simulink library "ddm"  (R2021b)
settings: Solver=VariableStepAuto  StartTime=0.0  StopTime=10.0  RelTol=1e-3
undefined symbols (not defined in the file or in its folder): ADDM_FrTMTqDev_X_Nm, ADDM_RrTMTqDev_X_Nm, ENUM_ADASACCSTA_ERROR, ENUM_ADASACCSTA_OFF, ENUM_ADASACCSTA_STANDBY, ENUM_ALLOWMOV_ALLOWREADY, ENUM_APS, ENUM_BRKSTA_ERROR, ENUM_BRKSTA_OFF, ENUM_BRKSTA_ON, ENUM_BRKSW_INVALID, ENUM_BRKSW_OFF, ENUM_BRKSW_ON, ENUM_CHGPREACTERRSTA_OBCPRE, ENUM_DCDCFAULTSTA_ANYFAULTLV1, ENUM_DCDCFAULTSTA_ANYFAULTLV2, ENUM_DRIVETRAIN_AWD, ENUM_DRIVETRAIN_FWD, ENUM_DRIVETRAIN_RWD, ENUM_EDUDRTSTA_NORMAL, ENUM_EPBSTA_APPLIED, ENUM_EPBSTA_RELEASED, ENUM_GEARACTUALPOSN_INVALID, ENUM_GEARACTUALPOSN_P, ENUM_HVBATTREADYPRE_READY, ENUM_MCUWARN_LV0, ENUM_MCUWARN_LV1, ENUM_MCUWARN_LV2, ENUM_MCUWARN_LV3, ENUM_MCUWARN_NOERROR, ENUM_OBCFAULTSTA_ANYFAULT, ENUM_PAS_R2F2, ENUM_PDFAULT_BATTPDFAIL, ENUM_PDFAULT_DCDCDISABLE, ENUM_PDFAULT_MCUDISABLE, ENUM_PDFAULT_MCUDISCHRG, ENUM_POWERSTA_OFF, ENUM_POWERSTA_ON, ENUM_POWERSTA_READY, ENUM_POWERSTA_STANDBY, ENUM_PRESSINDI_LOW, ENUM_PUFAULT_BATTUPFAIL, ENUM_PUFAULT_DCDCENABLEFAIL, ENUM_PUFAULT_PRECHRGCHKFAIL, ENUM_PUFAULT_SAFETYCHKFAIL, ENUM_PUSTATE_COMPLETED, ENUM_PWRSTASW_OFF, ENUM_PWRSTASW_OFFA, ENUM_PWRSTASW_OFFCHVCHRG, ENUM_PWRSTASW_OFFCLVCHRG, ENUM_PWRSTASW_ON, ENUM_PWRSTASW_ONHVCHRG, ENUM_PWRSTASW_READY, ENUM_PWRSTASW_STANDBY, ENUM_SHIFTCOMMAND_P, ENUM_SHIFTERERRSTA_PBUTTONFAILURE, ENUM_VEHMALFUNLV_2ND, ENUM_VEHMALFUNLV_3RD, ENUM_VEHMALFUNLV_4TH, ENUM_VEHMALFUNLV_NORMAL ... (+459)
libraries: hcu_lib x515, simulink x3
(part 4 of 25)

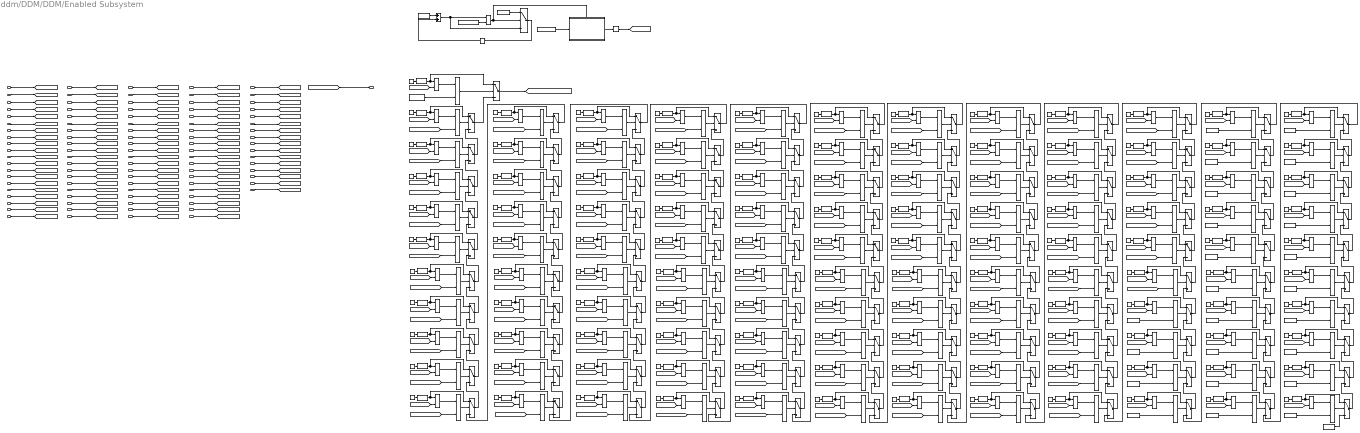
== system ddm/DDM/DDM/Enabled Subsystem ==
  VDDM_5vAPS1OoRCFS_flg : Inport
  VDDM_5vAPS2OoRCFS_flg : Inport  Port=2
  VDDM_BMSRdyCFS_flg : Inport  Port=3
  VDDM_BrkSWErrCFS_flg : Inport  Port=4
  VDDM_BrkSWNoBacCFS_flg : Inport  Port=5
  VDDM_C1ABM1CSCFS_flg : Inport  Port=6
  VDDM_C1ABM1LCCFS_flg : Inport  Port=7
  VDDM_C1ABM1RCCFS_flg : Inport  Port=8
  VDDM_C3BMS1CSCFS_flg : Inport  Port=9
  VDDM_C3BMS1LCCFS_flg : Inport  Port=10
  VDDM_C3BMS1RCCFS_flg : Inport  Port=11
  VDDM_C3BMS6CSCFS_flg : Inport  Port=12
  VDDM_C3BMS6LCCFS_flg : Inport  Port=13
  VDDM_C3BMS6RCCFS_flg : Inport  Port=14
  VDDM_C3CCU1CSCFS_flg : Inport  Port=15
  VDDM_C3CCU1LCCFS_flg : Inport  Port=16
  VDDM_C3CCU1RCCFS_flg : Inport  Port=17
  VDDM_C3CCU2CSCFS_flg : Inport  Port=18
  VDDM_C3CCU2LCCFS_flg : Inport  Port=19
  VDDM_C3CCU2RCCFS_flg : Inport  Port=20
  VDDM_DCDC4PreCFS_flg : Inport  Port=21
  VDDM_DCDCDisCFS_flg : Inport  Port=22
  VDDM_DCDCEnaCFS_flg : Inport  Port=23
  VDDM_DrStSWCFS_flg : Inport  Port=24
  VDDM_EPBLockTOCFS_flg : Inport  Port=25
  VDDM_EPBUnlockTOCFS_flg : Inport  Port=26
  VDDM_ESC1CSErrCFS_flg : Inport  Port=27
  VDDM_ESC1NoComCFS_flg : Inport  Port=28
  VDDM_ESC1RCErrCFS_flg : Inport  Port=29
  VDDM_ESC5CSErrCFS_flg : Inport  Port=30
  VDDM_ESC5NoComCFS_flg : Inport  Port=31
  VDDM_ESC5RCErrCFS_flg : Inport  Port=32
  VDDM_FLDoorSWCFS_flg : Inport  Port=33
  VDDM_FRDoorSWCFS_flg : Inport  Port=34
  VDDM_HVB4PreCFS_flg : Inport  Port=35
  VDDM_HVRlyCloCFS_flg : Inport  Port=36
  VDDM_HVRlyOpCFS_flg : Inport  Port=37
  VDDM_HiLvSaChkCFS_flg : Inport  Port=38
  VDDM_IniLVLoCFS_flg : Inport  Port=39
  VDDM_KeyAuthCFS_flg : Inport  Port=40
  VDDM_LVInErrCFS_flg : Inport  Port=41
  VDDM_LVSupHiCFS_flg : Inport  Port=42
  VDDM_LVSupLoCFS_flg : Inport  Port=43
  VDDM_Lv1ErrCFS_flg : Inport  Port=44
  VDDM_Lv2ErrCFS_flg : Inport  Port=45
  VDDM_Lv3ErrCFS_flg : Inport  Port=46
  VDDM_Lv4ErrCFS_flg : Inport  Port=47
  VDDM_MCU4PreCFS_flg : Inport  Port=48
  VDDM_MCUActCFS_flg : Inport  Port=49
  VDDM_MCUDisCFS_flg : Inport  Port=50
  VDDM_MCUNF1CSErrCFS_flg : Inport  Port=51
  VDDM_MCUNF1NoComCFS_flg : Inport  Port=52
  VDDM_MCUNF1RCErrCFS_flg : Inport  Port=53
  VDDM_MCUNR1CSErrCFS_flg : Inport  Port=54
  VDDM_MCUNR1NoComCFS_flg : Inport  Port=55
  VDDM_MCUNR1RCErrCFS_flg : Inport  Port=56
  VDDM_MidLvSaChkCFS_flg : Inport  Port=57
  VDDM_OBC4PreCFS_flg : Inport  Port=58
  VDDM_ONtoRdyCFS_flg : Inport  Port=59
  VDDM_RLDoorSWCFS_flg : Inport  Port=60
  VDDM_RRDoorSWCFS_flg : Inport  Port=61
  VDDM_Shifter1CSErrCFS_flg : Inport  Port=62
  VDDM_Shifter1NoComCFS_flg : Inport  Port=63
  VDDM_Shifter1RCErrCFS_flg : Inport  Port=64
  VDDM_HoodSWCFS_flg : Inport  Port=65
  VDDM_TailgaSWCFS_flg : Inport  Port=66
  VINP_ZoneDrMalfunLevel_enum : Inport  Port=67
  ZoneFrMalfunLevel_enum : Inport  Port=68
  VDDM_APS1SigOoRCFS_flg : Inport  Port=69
  VDDM_APS2SigOoRCFS_flg : Inport  Port=70
  VDDM_APSCorrErrCFS_flg : Inport  Port=71
  VDDM_FCM1NoComCFS_flg : Inport  Port=72
  VDDM_FCM1RCErrCFS_flg : Inport  Port=73
  VDDM_FCM1CSErrCFS_flg : Inport  Port=74
  VDDM_BMSSigErrCFS_flg : Inport  Port=75
  VDDM_FCMACCSigErrCFS_flg : Inport  Port=76
  VDDM_CCUSigErrCFS_flg : Inport  Port=77
  VDDM_ACCAccelCmdErrCFS_flg : Inport  Port=78
  VDDM_ESCSigErrCFS_flg : Inport  Port=79
  VDDM_ShifterSigErrCFS_flg : Inport  Port=80
  VDDM_DrVCUNoComCFS_flg : Inport  Port=81
  VDDM_FrVCUNoComCFS_flg : Inport  Port=82
  VDDM_ZoneDrSigErrCFS_flg : Inport  Port=83
  VDDM_ZoneFrSigErrCFS_flg : Inport  Port=84
  VDDM_EPS1NoComCFS_flg : Inport  Port=85
  VDDM_EPS1RCErrCFS_flg : Inport  Port=86
  VDDM_EPS1CSErrCFS_flg : Inport  Port=87
  VDDM_EPSSigErrCFS_flg : Inport  Port=88
  VDDM_FrMCUSigErrCFS_flg : Inport  Port=89
  VDDM_RrMCUSigErrCFS_flg : Inport  Port=90
  VDDM_EPB1NoComCFS_flg : Inport  Port=91
  VDDM_EPB1RCErrCFS_flg : Inport  Port=92
  VDDM_EPB1CSErrCFS_flg : Inport  Port=93
  VDDM_EPBSigErrCFS_flg : Inport  Port=94
  VDDM_FrMCUNTqErrCFS_flg : Inport  Port=95
  VDDM_RrMCUNTqErrCFS_flg : Inport  Port=96
  Add : Sum
  Constant : Constant  Value=ZERO_INT
  Constant1 : Constant  Value=ONE_INT
  Constant10 : Constant  Value=6  OutDataTypeStr=single
  Constant100 : Constant  Value=92  OutDataTypeStr=single
  Constant101 : Constant  Value=93  OutDataTypeStr=single
  Constant102 : Constant  Value=94  OutDataTypeStr=single
  Constant103 : Constant  Value=91  OutDataTypeStr=single
  Constant104 : Constant  Value=95  OutDataTypeStr=single
  Constant105 : Constant  Value=102  OutDataTypeStr=single
  Constant106 : Constant  Value=103  OutDataTypeStr=single
  Constant107 : Constant  Value=104  OutDataTypeStr=single
  Constant108 : Constant  Value=101  OutDataTypeStr=single
  Constant109 : Constant  Value=105  OutDataTypeStr=single
  Constant11 : Constant  Value=7  OutDataTypeStr=single
  Constant110 : Constant  Value=106  OutDataTypeStr=single
  Constant111 : Constant  Value=107  OutDataTypeStr=single
  Constant112 : Constant  Value=108  OutDataTypeStr=single
  Constant113 : Constant  Value=109  OutDataTypeStr=single
  Constant114 : Constant  Value=110  OutDataTypeStr=single
  Constant115 : Constant  Value=112  OutDataTypeStr=single
  Constant116 : Constant  Value=113  OutDataTypeStr=single
  Constant117 : Constant  Value=114  OutDataTypeStr=single
  Constant118 : Constant  Value=111  OutDataTypeStr=single
  Constant119 : Constant  Value=115  OutDataTypeStr=single
  Constant12 : Constant  Value=8  OutDataTypeStr=single
  Constant120 : Constant  Value=116  OutDataTypeStr=single
  Constant121 : Constant  Value=117  OutDataTypeStr=single
  Constant122 : Constant  Value=118  OutDataTypeStr=single
  Constant123 : Constant  Value=119  OutDataTypeStr=single
  Constant124 : Constant  Value=120  OutDataTypeStr=single
  Constant{125..132,135..150} (24 alike) : Constant  Value=FALSE
  Constant13 : Constant  Value=9  OutDataTypeStr=single
  Constant133 : Constant  Value=ZERO_INT
  Constant134 : Constant  Value=KDDM_DTCClockerMax_cnt
  Constant14 : Constant  Value=10  OutDataTypeStr=single
  Constant15 : Constant  Value=16  OutDataTypeStr=single
  Constant16 : Constant  Value=17  OutDataTypeStr=single
  Constant17 : Constant  Value=18  OutDataTypeStr=single
  Constant18 : Constant  Value=19  OutDataTypeStr=single
  Constant19 : Constant  Value=20  OutDataTypeStr=single
  Constant2 : Constant  Value=2  OutDataTypeStr=single
  Constant20 : Constant  Value=12  OutDataTypeStr=single
  Constant21 : Constant  Value=13  OutDataTypeStr=single
  Constant22 : Constant  Value=14  OutDataTypeStr=single
  Constant23 : Constant  Value=11  OutDataTypeStr=single
  Constant24 : Constant  Value=15  OutDataTypeStr=single
  Constant25 : Constant  Value=26  OutDataTypeStr=single
  Constant26 : Constant  Value=27  OutDataTypeStr=single
  Constant27 : Constant  Value=28  OutDataTypeStr=single
  Constant28 : Constant  Value=29  OutDataTypeStr=single
  Constant29 : Constant  Value=30  OutDataTypeStr=single
  Constant3 : Constant  Value=3  OutDataTypeStr=single
  Constant30 : Constant  Value=22  OutDataTypeStr=single
  Constant31 : Constant  Value=23  OutDataTypeStr=single
  Constant32 : Constant  Value=24  OutDataTypeStr=single
  Constant33 : Constant  Value=21  OutDataTypeStr=single
  Constant34 : Constant  Value=25  OutDataTypeStr=single
  Constant35 : Constant  Value=36  OutDataTypeStr=single
  Constant36 : Constant  Value=37  OutDataTypeStr=single
  Constant37 : Constant  Value=38  OutDataTypeStr=single
  Constant38 : Constant  Value=39  OutDataTypeStr=single
  Constant39 : Constant  Value=40  OutDataTypeStr=single
  Constant4 : Constant  Value=TRUE
  Constant40 : Constant  Value=32  OutDataTypeStr=single
  Constant41 : Constant  Value=33  OutDataTypeStr=single
  Constant42 : Constant  Value=34  OutDataTypeStr=single
  Constant43 : Constant  Value=31  OutDataTypeStr=single
  Constant44 : Constant  Value=35  OutDataTypeStr=single
  Constant45 : Constant  Value=46  OutDataTypeStr=single
  Constant46 : Constant  Value=47  OutDataTypeStr=single
  Constant47 : Constant  Value=48  OutDataTypeStr=single
  Constant48 : Constant  Value=49  OutDataTypeStr=single
  Constant49 : Constant  Value=50  OutDataTypeStr=single
  Constant5 : Constant  Value=KDDM_DTCDelay_cnt
  Constant50 : Constant  Value=42  OutDataTypeStr=single
  Constant51 : Constant  Value=43  OutDataTypeStr=single
  Constant52 : Constant  Value=44  OutDataTypeStr=single
  Constant53 : Constant  Value=41  OutDataTypeStr=single
  Constant54 : Constant  Value=45  OutDataTypeStr=single
  Constant55 : Constant  Value=56  OutDataTypeStr=single
  Constant56 : Constant  Value=57  OutDataTypeStr=single
  Constant57 : Constant  Value=58  OutDataTypeStr=single
  Constant58 : Constant  Value=59  OutDataTypeStr=single
  Constant59 : Constant  Value=60  OutDataTypeStr=single
  Constant6 : Constant  Value=4  OutDataTypeStr=single
  Constant60 : Constant  Value=52  OutDataTypeStr=single
  Constant61 : Constant  Value=53  OutDataTypeStr=single
  Constant62 : Constant  Value=54  OutDataTypeStr=single
  Constant63 : Constant  Value=51  OutDataTypeStr=single
  Constant64 : Constant  Value=55  OutDataTypeStr=single
  Constant65 : Constant  Value=66  OutDataTypeStr=single
  Constant66 : Constant  Value=67  OutDataTypeStr=single
  Constant67 : Constant  Value=68  OutDataTypeStr=single
  Constant68 : Constant  Value=69  OutDataTypeStr=single
  Constant69 : Constant  Value=70  OutDataTypeStr=single
  Constant7 : Constant  OutDataTypeStr=single
  Constant70 : Constant  Value=62  OutDataTypeStr=single
  Constant71 : Constant  Value=63  OutDataTypeStr=single
  Constant72 : Constant  Value=64  OutDataTypeStr=single
  Constant73 : Constant  Value=61  OutDataTypeStr=single
  Constant74 : Constant  Value=65  OutDataTypeStr=single
  Constant75 : Constant  Value=76  OutDataTypeStr=single
  Constant76 : Constant  Value=77  OutDataTypeStr=single
  Constant77 : Constant  Value=78  OutDataTypeStr=single
  Constant78 : Constant  Value=79  OutDataTypeStr=single
  Constant79 : Constant  Value=80  OutDataTypeStr=single
  Constant8 : Constant  Value=5  OutDataTypeStr=single
  Constant80 : Constant  Value=72  OutDataTypeStr=single
  Constant81 : Constant  Value=73  OutDataTypeStr=single
  Constant82 : Constant  Value=74  OutDataTypeStr=single
  Constant83 : Constant  Value=71  OutDataTypeStr=single
  Constant84 : Constant  Value=75  OutDataTypeStr=single
  Constant85 : Constant  Value=86  OutDataTypeStr=single
  Constant86 : Constant  Value=87  OutDataTypeStr=single
  Constant87 : Constant  Value=88  OutDataTypeStr=single
  Constant88 : Constant  Value=89  OutDataTypeStr=single
  Constant89 : Constant  Value=90  OutDataTypeStr=single
  Constant9 : Constant  Value=0  OutDataTypeStr=uint8
  Constant90 : Constant  Value=82  OutDataTypeStr=single
  Constant91 : Constant  Value=83  OutDataTypeStr=single
  Constant92 : Constant  Value=84  OutDataTypeStr=single
  Constant93 : Constant  Value=81  OutDataTypeStr=single
  Constant94 : Constant  Value=85  OutDataTypeStr=single
  Constant95 : Constant  Value=96  OutDataTypeStr=single
  Constant96 : Constant  Value=97  OutDataTypeStr=single
  Constant97 : Constant  Value=98  OutDataTypeStr=single
  Constant98 : Constant  Value=99  OutDataTypeStr=single
  Constant99 : Constant  Value=100  OutDataTypeStr=single
  Data Type Conversion{,1..120} (121 alike) : DataTypeConversion  OutDataTypeStr=uint8
  Delay : Delay  DelayLength=1
  IC : InitialCondition  Value=0
  Logical Operator{,1..120} (121 alike) : Logic  AllPortsSameDT=off  OutDataTypeStr=boolean
  Relational Operator : RelationalOperator  Operator=>  OutDataTypeStr=boolean  RndMeth=Simplest
  Relational Operator{1..121} (121 alike) : RelationalOperator  Operator===  OutDataTypeStr=boolean  RndMeth=Simplest
  Subsystem : Subsystem
  Switch{,1..121} (122 alike) : Switch  Criteria=u2 > Threshold
  VDDM_DTCDetect_enum : Outport
  wires:
  Constant1/1 -> Add/1
  IC/1 -> [DTC_clocker]
  Constant/1 -> Switch/1
  Subsystem/1(VDDM_DTCCounter_cnt) -> IC/1
  Add/1 -> Relational Operator/1, Switch/3
  Switch/1 -> Delay/1
  Delay/1 -> Add/2
  Constant134/1 -> Subsystem/1(KDDM_DTCClockerMax_cnt)
  Relational Operator/1 -> Switch/2, Subsystem/Trigger
  Constant5/1 -> Relational Operator/2
  Relational Operator13/1 -> Logical Operator20/1
  Constant16/1 -> Data Type Conversion18/1
  Switch1/1 -> [VDDM_DTCDetect_enum]  "VDDM_DTCDetect_enum"
  Relational Operator16/1 -> Logical Operator14/1
  [DTC_clocker] -> Relational Operator16/2
  Data Type Conversion16/1 -> Relational Operator18/1, Switch18/1
  Constant22/1 -> Data Type Conversion15/1
  Data Type Conversion18/1 -> Relational Operator20/1, Switch20/1
  Logical Operator16/1 -> Switch18/2
  Constant11/1 -> Data Type Conversion7/1
  Switch6/1 -> Switch5/3
  Switch16/1 -> Switch15/3
  [DTC_clocker] -> Relational Operator21/2
  Relational Operator14/1 -> Logical Operator12/1
  [VDDM_C3CCU2RCCFS_flg] -> Logical Operator12/2
  [DTC_clocker] -> Relational Operator19/2
  Relational Operator19/1 -> Logical Operator17/1
  Switch19/1 -> Switch18/3
  Constant20/1 -> Data Type Conversion13/1
  Constant15/1 -> Data Type Conversion17/1
  Logical Operator11/1 -> Switch14/2
  Switch15/1 -> Switch14/3
  Data Type Conversion6/1 -> Relational Operator7/1, Switch7/1
  [DTC_clocker] -> Relational Operator11/2
  [VDDM_C1ABM1LCCFS_flg] -> Logical Operator7/2
  Logical Operator10/1 -> Switch11/2
  [DTC_clocker] -> Relational Operator10/2
  Switch9/1 -> Switch8/3
  Switch10/1 -> Switch9/3
  Switch8/1 -> Switch7/3
  Logical Operator9/1 -> Switch10/2
  [DTC_clocker] -> Relational Operator7/2
  [DTC_clocker] -> Relational Operator5/2
  Switch3/1 -> Switch2/3
  [DTC_clocker] -> Relational Operator6/2
  Data Type Conversion4/1 -> Relational Operator5/1, Switch5/1
  Constant8/1 -> Data Type Conversion5/1
  Logical Operator/1 -> Switch2/2
  [DTC_clocker] -> Relational Operator1/2
  Relational Operator1/1 -> Logical Operator/1
  Data Type Conversion2/1 -> Relational Operator2/1, Switch3/1
  Constant4/1 -> Logical Operator1/2
  Logical Operator1/1 -> Switch1/2
  Data Type Conversion8/1 -> Relational Operator9/1, Switch9/1
  Relational Operator29/1 -> Logical Operator27/1
  Relational Operator27/1 -> Logical Operator25/1
  [VDDM_EPBUnlockTOCFS_flg] -> Logical Operator27/2
  Switch26/1 -> Switch25/3
  [DTC_clocker] -> Relational Operator29/2
  Switch7/1 -> Switch6/3
  Switch28/1 -> Switch27/3
  Data Type Conversion28/1 -> Relational Operator30/1, Switch30/1
  Switch22/1 -> Switch31/3
  Constant27/1 -> Data Type Conversion29/1
  Constant26/1 -> Data Type Conversion28/1
  Data Type Conversion15/1 -> Relational Operator17/1, Switch17/1
  Logical Operator26/1 -> Switch28/2
  [VDDM_C3BMS6LCCFS_flg] -> Logical Operator14/2
  Switch14/1 -> Switch11/3
  Relational Operator32/1 -> Logical Operator31/1
  Switch63/1 -> Switch62/3
  [VDDM_MCUNR1NoComCFS_flg] -> Logical Operator56/2
  Relational Operator59/1 -> Logical Operator57/1
  Data Type Conversion17/1 -> Relational Operator19/1, Switch19/1
  Relational Operator74/1 -> Logical Operator72/1
  Switch69/1 -> Switch68/3
  [DTC_clocker] -> Relational Operator47/2
  [DTC_clocker] -> Relational Operator76/2
  Relational Operator73/1 -> Logical Operator80/1
  Constant17/1 -> Data Type Conversion19/1
  Constant65/1 -> Data Type Conversion67/1
  [VDDM_FCM1NoComCFS_flg] -> Logical Operator73/2
  Switch74/1 -> Switch63/3
  [VDDM_C1ABM1RCCFS_flg] -> Logical Operator8/2
  [VDDM_ESC1RCErrCFS_flg] -> Logical Operator30/2
  Switch11/1 -> Switch10/3
  Data Type Conversion71/1 -> Relational Operator72/1, Switch74/1
  Relational Operator44/1 -> Logical Operator42/1
  Constant67/1 -> Data Type Conversion69/1
  Logical Operator3/1 -> Switch4/2
  [VDDM_MCUNF1CSErrCFS_flg] -> Logical Operator51/2
  Data Type Conversion58/1 -> Relational Operator60/1, Switch60/1
  Constant71/1 -> Data Type Conversion64/1
  Data Type Conversion66/1 -> Relational Operator68/1, Switch68/1
  Data Type Conversion23/1 -> Relational Operator25/1, Switch25/1
  Relational Operator24/1 -> Logical Operator22/1
  Relational Operator65/1 -> Logical Operator63/1
  Relational Operator71/1 -> Logical Operator69/1
  Logical Operator69/1 -> Switch71/2
  Switch62/1 -> Switch71/3
  Relational Operator70/1 -> Logical Operator68/1
  Switch65/1 -> Switch64/3
  Data Type Conversion53/1 -> Relational Operator55/1, Switch55/1
  [DTC_clocker] -> Relational Operator30/2
  Data Type Conversion12/1 -> Relational Operator14/1, Switch13/1
  [VINP_ZoneDrMalfunLevel_enum] -> Logical Operator68/2
  Constant73/1 -> Data Type Conversion61/1
  Relational Operator63/1 -> Logical Operator70/1
  Data Type Conversion51/1 -> Relational Operator52/1, Switch54/1
  Data Type Conversion61/1 -> Relational Operator62/1, Switch64/1
  Constant28/1 -> Data Type Conversion30/1
  Logical Operator68/1 -> Switch70/2
  Constant63/1 -> Data Type Conversion51/1
  Logical Operator58/1 -> Switch60/2
  Constant82/1 -> Data Type Conversion75/1
  [VDDM_MCUNF1RCErrCFS_flg] -> Logical Operator54/2
  Constant74/1 -> Data Type Conversion66/1
  Logical Operator27/1 -> Switch29/2
  [DTC_clocker] -> Relational Operator58/2
  Logical Operator52/1 -> Switch53/2
  Data Type Conversion54/1 -> Relational Operator56/1, Switch56/1
  Logical Operator54/1 -> Switch56/2
  Constant48/1 -> Data Type Conversion50/1
  Logical Operator60/1 -> Switch52/2
  Constant19/1 -> Data Type Conversion12/1
  Data Type Conversion26/1 -> Relational Operator28/1, Switch28/1
  [VDDM_HiLvSaChkCFS_flg] -> Logical Operator39/2
  [DTC_clocker] -> Relational Operator8/2
  Relational Operator57/1 -> Logical Operator55/1
  Switch31/1 -> Switch30/3
  [DTC_clocker] -> Relational Operator54/2
  [DTC_clocker] -> Relational Operator49/2
  [DTC_clocker] -> Relational Operator17/2
  Logical Operator47/1 -> Switch49/2
  Data Type Conversion41/1 -> Relational Operator42/1, Switch44/1
  [DTC_clocker] -> Relational Operator51/2
  [VDDM_LVInErrCFS_flg] -> Logical Operator41/2
  Relational Operator50/1 -> Logical Operator48/1
  Constant45/1 -> Data Type Conversion47/1
  Relational Operator6/1 -> Logical Operator5/1
  Switch80/1 -> Switch79/3
  [DTC_clocker] -> Relational Operator50/2
  Logical Operator2/1 -> Switch3/2
  Data Type Conversion43/1 -> Relational Operator45/1, Switch45/1
  Constant51/1 -> Data Type Conversion44/1
  Logical Operator17/1 -> Switch19/2
  Logical Operator64/1 -> Switch66/2
  Switch44/1 -> Switch33/3
  Switch42/1 -> Switch51/3
  Constant52/1 -> Data Type Conversion45/1
  Constant3/1 -> Data Type Conversion3/1
  Data Type Conversion44/1 -> Relational Operator46/1, Switch46/1
  Switch46/1 -> Switch45/3
  Constant49/1 -> Data Type Conversion42/1
  [VDDM_APS2SigOoRCFS_flg] -> Logical Operator62/2
  [VDDM_MCUActCFS_flg] -> Logical Operator50/2
  Logical Operator44/1 -> Switch46/2
  [VDDM_LVSupLoCFS_flg] -> Logical Operator44/2
  [DTC_clocker] -> Relational Operator66/2
  Relational Operator48/1 -> Logical Operator46/1
  Data Type Conversion7/1 -> Relational Operator8/1, Switch8/1
  [DTC_clocker] -> Relational Operator45/2
  [VDDM_C3CCU1CSCFS_flg] -> Logical Operator16/2
  [VDDM_MCUDisCFS_flg] -> Logical Operator42/2
  Constant18/1 -> Data Type Conversion20/1
  Data Type Conversion32/1 -> Relational Operator34/1, Switch33/1
  Data Type Conversion19/1 -> Relational Operator21/1, Switch21/1
  Constant2/1 -> Data Type Conversion2/1
  Switch50/1 -> Switch49/3
  [VDDM_OBC4PreCFS_flg] -> Logical Operator59/2
  [DTC_clocker] -> Relational Operator32/2
  Logical Operator46/1 -> Switch48/2
  [VDDM_ESC1CSErrCFS_flg] -> Logical Operator28/2
  Constant78/1 -> Data Type Conversion80/1
  [DTC_clocker] -> Relational Operator36/2
  [VDDM_HVRlyOpCFS_flg] -> Logical Operator38/2
  Data Type Conversion39/1 -> Relational Operator41/1, Switch41/1
  Logical Operator32/1 -> Switch33/2
  Constant41/1 -> Data Type Conversion34/1
  Constant47/1 -> Data Type Conversion49/1
  Logical Operator22/1 -> Switch23/2
  Logical Operator40/1 -> Switch32/2
  Relational Operator34/1 -> Logical Operator32/1
  Logical Operator45/1 -> Switch47/2
  Constant36/1 -> Data Type Conversion38/1
  Data Type Conversion50/1 -> Relational Operator43/1, Switch42/1
  Relational Operator38/1 -> Logical Operator36/1
  Constant44/1 -> Data Type Conversion36/1
  Data Type Conversion42/1 -> Relational Operator44/1, Switch43/1
  Constant37/1 -> Data Type Conversion39/1
  [DTC_clocker] -> Relational Operator43/2
  Constant38/1 -> Data Type Conversion40/1
  Switch39/1 -> Switch38/3
  Constant6/1 -> Data Type Conversion4/1
  Logical Operator35/1 -> Switch37/2
  Logical Operator39/1 -> Switch41/2
  [DTC_clocker] -> Relational Operator72/2
  [DTC_clocker] -> Relational Operator40/2
  Switch32/1 -> Switch41/3
  [VDDM_MCU4PreCFS_flg] -> Logical Operator49/2
  Data Type Conversion3/1 -> Relational Operator4/1, Switch4/1
  Constant25/1 -> Data Type Conversion27/1
  Data Type Conversion33/1 -> Relational Operator35/1, Switch35/1
  Logical Operator31/1 -> Switch34/2
  Switch45/1 -> Switch44/3
  Switch5/1 -> Switch4/3
  Logical Operator20/1 -> Switch12/2
  [DTC_clocker] -> Relational Operator27/2
  Switch27/1 -> Switch26/3
  [DTC_clocker] -> Relational Operator37/2
  [DTC_clocker] -> Relational Operator41/2
  Relational Operator36/1 -> Logical Operator34/1
  [VDDM_ESC5RCErrCFS_flg] -> Logical Operator33/2
  Switch101/1 -> Switch100/3
  [DTC_clocker] -> Relational Operator92/2
  [VDDM_Shifter1CSErrCFS_flg] -> Logical Operator63/2
  Relational Operator52/1 -> Logical Operator51/1
  Logical Operator94/1 -> Switch96/2
  [DTC_clocker] -> Relational Operator101/2
  [VDDM_EPBSigErrCFS_flg] -> Logical Operator95/2
  Constant69/1 -> Data Type Conversion62/1
  Relational Operator83/1 -> Logical Operator90/1
  [DTC_clocker] -> Relational Operator70/2
  Data Type Conversion100/1 -> Relational Operator93/1, Switch92/1
  [DTC_clocker] -> Relational Operator94/2
  Data Type Conversion57/1 -> Relational Operator59/1, Switch59/1
  Data Type Conversion20/1 -> Relational Operator13/1, Switch12/1
  Relational Operator49/1 -> Logical Operator47/1
  Switch53/1 -> Switch52/3
  [VDDM_RrMCUNTqErrCFS_flg] -> Logical Operator97/2
  Relational Operator95/1 -> Logical Operator93/1
  Constant88/1 -> Data Type Conversion90/1
  Relational Operator101/1 -> Logical Operator99/1
  [VDDM_RRDoorSWCFS_flg] -> Logical Operator61/2
  Constant23/1 -> Data Type Conversion11/1
  Relational Operator94/1 -> Logical Operator92/1
  Switch54/1 -> Switch43/3
  [DTC_clocker] -> Relational Operator63/2
  [DTC_clocker] -> Relational Operator42/2
  [DTC_clocker] -> Relational Operator98/2
  Logical Operator4/1 -> Switch5/2
  Logical Operator92/1 -> Switch93/2
  Data Type Conversion/1 -> Relational Operator3/1, Switch1/1
  Relational Operator92/1 -> Logical Operator91/1
  Constant98/1 -> Data Type Conversion100/1
  Logical Operator33/1 -> Switch35/2
  Switch48/1 -> Switch47/3
  Data Type Conversion81/1 -> Relational Operator82/1, Switch84/1
  Constant101/1 -> Data Type Conversion94/1
  Constant54/1 -> Data Type Conversion46/1
  Data Type Conversion84/1 -> Relational Operator86/1, Switch86/1
  Switch94/1 -> Switch83/3
  [DTC_clocker] -> Relational Operator56/2
  Constant13/1 -> Data Type Conversion9/1
  Constant85/1 -> Data Type Conversion87/1
  Switch23/1 -> Switch22/3
  [DTC_clocker] -> Relational Operator26/2
  Switch92/1 -> Switch101/3
  Switch89/1 -> Switch88/3
  Data Type Conversion73/1 -> Relational Operator75/1, Switch75/1
  [VDDM_HVRlyCloCFS_flg] -> Logical Operator37/2
  Data Type Conversion27/1 -> Relational Operator29/1, Switch29/1
  Logical Operator86/1 -> Switch88/2
  Constant81/1 -> Data Type Conversion74/1
  Data Type Conversion14/1 -> Relational Operator16/1, Switch16/1
  [VDDM_ONtoRdyCFS_flg] -> Logical Operator60/2
  Switch71/1 -> Switch70/3
  Switch87/1 -> Switch86/3
  [DTC_clocker] -> Relational Operator85/2
  Data Type Conversion70/1 -> Relational Operator63/1, Switch62/1
  Relational Operator82/1 -> Logical Operator81/1
  Logical Operator83/1 -> Switch85/2
  Relational Operator78/1 -> Logical Operator76/1
  [DTC_clocker] -> Relational Operator86/2
  Data Type Conversion35/1 -> Relational Operator37/1, Switch37/1
  Relational Operator12/1 -> Logical Operator11/1
  Constant56/1 -> Data Type Conversion58/1
  Constant90/1 -> Data Type Conversion83/1
  Relational Operator15/1 -> Logical Operator13/1
  Data Type Conversion82/1 -> Relational Operator84/1, Switch83/1
  [VDDM_MCUNF1NoComCFS_flg] -> Logical Operator53/2
  [VDDM_DCDC4PreCFS_flg] -> Logical Operator21/2
  Constant93/1 -> Data Type Conversion81/1
  Logical Operator55/1 -> Switch57/2
  Data Type Conversion93/1 -> Relational Operator95/1, Switch95/1
  Switch83/1 -> Switch82/3
  Logical Operator85/1 -> Switch87/2
  [DTC_clocker] -> Relational Operator69/2
  Switch29/1 -> Switch28/3
  Switch70/1 -> Switch69/3
  Constant87/1 -> Data Type Conversion89/1
  [DTC_clocker] -> Relational Operator84/2
  [DTC_clocker] -> Relational Operator87/2
  Switch38/1 -> Switch37/3
  Relational Operator11/1 -> Logical Operator10/1
  Relational Operator4/1 -> Logical Operator3/1
  Logical Operator88/1 -> Switch90/2
  Logical Operator76/1 -> Switch78/2
  Switch78/1 -> Switch77/3
  Relational Operator88/1 -> Logical Operator86/1
  Relational Operator89/1 -> Logical Operator87/1
  Switch43/1 -> Switch42/3
  Data Type Conversion34/1 -> Relational Operator36/1, Switch36/1
  [DTC_clocker] -> Relational Operator81/2
  [VDDM_EPS1NoComCFS_flg] -> Logical Operator86/2
  Relational Operator10/1 -> Logical Operator9/1
  Relational Operator72/1 -> Logical Operator71/1
  Relational Operator55/1 -> Logical Operator53/1
  Switch52/1 -> Switch61/3
  Constant39/1 -> Data Type Conversion32/1
  [VDDM_FrMCUNTqErrCFS_flg] -> Logical Operator96/2
  Constant89/1 -> Data Type Conversion82/1
  Logical Operator49/1 -> Switch51/2
  [VDDM_EPS1RCErrCFS_flg] -> Logical Operator87/2
  Relational Operator17/1 -> Logical Operator15/1
  Logical Operator6/1 -> Switch7/2
  [VDDM_FLDoorSWCFS_flg] -> Logical Operator34/2
  Relational Operator18/1 -> Logical Operator16/1
  [DTC_clocker] -> Relational Operator75/2
  Constant40/1 -> Data Type Conversion33/1
  Data Type Conversion68/1 -> Relational Operator70/1, Switch70/1
  [VDDM_ESCSigErrCFS_flg] -> Logical Operator80/2
  [DTC_clocker] -> Relational Operator59/2
  Constant75/1 -> Data Type Conversion77/1
  Data Type Conversion72/1 -> Relational Operator74/1, Switch73/1
  [VDDM_MCUNR1RCErrCFS_flg] -> Logical Operator57/2
  Data Type Conversion74/1 -> Relational Operator76/1, Switch76/1
  Switch88/1 -> Switch87/3
  [DTC_clocker] -> Relational Operator12/2
  [DTC_clocker] -> Relational Operator77/2
  [DTC_clocker] -> Relational Operator74/2
  Relational Operator111/1 -> Logical Operator108/1
  Switch68/1 -> Switch67/3
  Switch49/1 -> Switch48/3
  Constant147/1 -> Logical Operator109/2
  Relational Operator9/1 -> Logical Operator8/1
  [DTC_clocker] -> Relational Operator95/2
  Logical Operator105/1 -> Switch108/2
  Logical Operator77/1 -> Switch79/2
  [DTC_clocker] -> Relational Operator52/2
  Relational Operator102/1 -> Logical Operator109/1
  Relational Operator53/1 -> Logical Operator60/1
  [DTC_clocker] -> Relational Operator4/2
  Logical Operator62/1 -> Switch63/2
  Switch13/1 -> Switch12/3
  [VDDM_FrMCUSigErrCFS_flg] -> Logical Operator90/2
  Constant140/1 -> Logical Operator104/2
  Logical Operator75/1 -> Switch77/2
  Constant76/1 -> Data Type Conversion78/1
  Data Type Conversion65/1 -> Relational Operator67/1, Switch67/1
  [VDDM_C3CCU2LCCFS_flg] -> Logical Operator20/2
  [VDDM_DCDCDisCFS_flg] -> Logical Operator23/2
  Switch73/1 -> Switch72/3
  Switch90/1 -> Switch89/3
  Relational Operator105/1 -> Logical Operator101/1
  Relational Operator69/1 -> Logical Operator67/1
  Switch56/1 -> Switch55/3
  Data Type Conversion21/1 -> Relational Operator22/1, Switch24/1
  [DTC_clocker] -> Relational Operator28/2
  [VDDM_RrMCUSigErrCFS_flg] -> Logical Operator82/2
  Relational Operator93/1 -> Logical Operator100/1
  [VDDM_RLDoorSWCFS_flg] -> Logical Operator52/2
  Switch34/1 -> Switch23/3
  Switch106/1 -> Switch93/3
  Constant60/1 -> Data Type Conversion53/1
  Relational Operator28/1 -> Logical Operator26/1
  [DTC_clocker] -> Relational Operator62/2
  Logical Operator19/1 -> Switch21/2
  Relational Operator77/1 -> Logical Operator75/1
  Constant7/1 -> Data Type Conversion1/1
  Logical Operator70/1 -> Switch62/2
  Data Type Conversion91/1 -> Relational Operator92/1, Switch94/1
  [VDDM_HoodSWCFS_flg] -> Logical Operator66/2
  Data Type Conversion52/1 -> Relational Operator54/1, Switch53/1
  Switch100/1 -> Switch99/3
  [DTC_clocker] -> Relational Operator13/2
  Logical Operator53/1 -> Switch55/2
  Constant100/1 -> Data Type Conversion93/1
  Data Type Conversion76/1 -> Relational Operator78/1, Switch78/1
  Logical Operator59/1 -> Switch61/2
  Constant14/1 -> Data Type Conversion10/1
  Logical Operator30/1 -> Switch22/2
  Constant94/1 -> Data Type Conversion86/1
  Logical Operator97/1 -> Switch99/2
  [DTC_clocker] -> Relational Operator88/2
  [VDDM_HVB4PreCFS_flg] -> Logical Operator36/2
  Relational Operator99/1 -> Logical Operator97/1
  Relational Operator100/1 -> Logical Operator98/1
  [DTC_clocker] -> Relational Operator68/2
  Constant68/1 -> Data Type Conversion70/1
  [VDDM_MCUNR1CSErrCFS_flg] -> Logical Operator55/2
  Logical Operator111/1 -> Switch114/2
  Relational Operator25/1 -> Logical Operator23/1
  Constant110/1 -> Data Type Conversion108/1
  [VDDM_EPBLockTOCFS_flg] -> Logical Operator26/2
  Switch79/1 -> Switch78/3
  Logical Operator109/1 -> Switch102/2
  Switch81/1 -> Switch80/3
  Relational Operator113/1 -> Logical Operator120/1
  [DTC_clocker] -> Relational Operator61/2
  [DTC_clocker] -> Relational Operator33/2
  Relational Operator90/1 -> Logical Operator88/1
  Relational Operator2/1 -> Logical Operator2/1
  Relational Operator120/1 -> Logical Operator117/1
  Constant123/1 -> Data Type Conversion111/1
  Data Type Conversion29/1 -> Relational Operator31/1, Switch31/1
  Logical Operator74/1 -> Switch76/2
  Data Type Conversion11/1 -> Relational Operator12/1, Switch14/1
  Logical Operator21/1 -> Switch24/2
  Relational Operator114/1 -> Logical Operator112/1
  Relational Operator41/1 -> Logical Operator39/1
  Relational Operator85/1 -> Logical Operator83/1
  Relational Operator35/1 -> Logical Operator33/1
  Constant122/1 -> Data Type Conversion120/1
  [DTC_clocker] -> Relational Operator46/2
  Relational Operator5/1 -> Logical Operator4/1
  Data Type Conversion49/1 -> Relational Operator51/1, Switch51/1
  Relational Operator119/1 -> Logical Operator116/1
  Data Type Conversion106/1 -> Relational Operator109/1, Switch109/1
  Constant33/1 -> Data Type Conversion21/1
  Logical Operator23/1 -> Switch25/2
  [VDDM_ESC5NoComCFS_flg] -> Logical Operator31/2
  [VDDM_ESC5CSErrCFS_flg] -> Logical Operator22/2
  Data Type Conversion80/1 -> Relational Operator73/1, Switch72/1
  Switch57/1 -> Switch56/3
  [DTC_clocker] -> Relational Operator99/2
  [VDDM_EPS1CSErrCFS_flg] -> Logical Operator88/2
  [VDDM_C3BMS1LCCFS_flg] -> Logical Operator10/2
  Constant43/1 -> Data Type Conversion31/1
  Switch82/1 -> Switch91/3
  Switch114/1 -> Switch113/3
  Logical Operator78/1 -> Switch80/2
  Logical Operator119/1 -> Switch112/2
  [VDDM_ShifterSigErrCFS_flg] -> Logical Operator72/2
  Relational Operator37/1 -> Logical Operator35/1
  Relational Operator98/1 -> Logical Operator96/1
  [DTC_clocker] -> Relational Operator113/2
  Constant117/1 -> Data Type Conversion116/1
  [VDDM_C1ABM1CSCFS_flg] -> Logical Operator6/2
  [VDDM_FCM1RCErrCFS_flg] -> Logical Operator74/2
  Constant128/1 -> Logical Operator118/2
  Relational Operator76/1 -> Logical Operator74/1
  Logical Operator120/1 -> Switch113/2
  Switch112/1 -> Switch121/3
  Data Type Conversion87/1 -> Relational Operator89/1, Switch89/1
  [VDDM_BrkSWErrCFS_flg] -> Logical Operator4/2
  Logical Operator93/1 -> Switch95/2
  [VDDM_C3BMS1CSCFS_flg] -> Logical Operator9/2
  Logical Operator90/1 -> Switch82/2
  Relational Operator103/1 -> Logical Operator110/1
  Switch33/1 -> Switch32/3
  Constant53/1 -> Data Type Conversion41/1
  Switch105/1 -> Switch104/3
  Relational Operator20/1 -> Logical Operator18/1
  Logical Operator37/1 -> Switch39/2
  Data Type Conversion55/1 -> Relational Operator57/1, Switch57/1
  Constant115/1 -> Data Type Conversion114/1
  Constant62/1 -> Data Type Conversion55/1
  Constant92/1 -> Data Type Conversion85/1
  Constant64/1 -> Data Type Conversion56/1
  Data Type Conversion98/1 -> Relational Operator100/1, Switch100/1
  Switch108/1 -> Switch107/3
  Constant126/1 -> Logical Operator116/2
  Switch107/1 -> Switch106/3
  [DTC_clocker] -> Relational Operator14/2
  Data Type Conversion109/1 -> Relational Operator102/1, Switch102/1
  Switch59/1 -> Switch58/3
  Switch18/1 -> Switch17/3
  Data Type Conversion38/1 -> Relational Operator40/1, Switch40/1
  Relational Operator30/1 -> Logical Operator28/1
  Relational Operator112/1 -> Logical Operator119/1
  [VDDM_BMSRdyCFS_flg] -> Logical Operator3/2
  [DTC_clocker] -> Relational Operator93/2
  Switch35/1 -> Switch34/3
  Logical Operator114/1 -> Switch117/2
  [DTC_clocker] -> Relational Operator97/2
  Data Type Conversion69/1 -> Relational Operator71/1, Switch71/1
  Logical Operator82/1 -> Switch83/2
  Logical Operator98/1 -> Switch100/2
  Data Type Conversion86/1 -> Relational Operator88/1, Switch88/1
  Constant141/1 -> Logical Operator114/2
  Constant137/1 -> Logical Operator100/2
  Switch60/1 -> Switch59/3
  Relational Operator45/1 -> Logical Operator43/1
  Data Type Conversion111/1 -> Relational Operator115/1, Switch114/1
  Switch41/1 -> Switch40/3
  Switch2/1 -> Switch1/3
  Constant12/1 -> Data Type Conversion8/1
  [VDDM_EPB1CSErrCFS_flg] -> Logical Operator94/2
  Data Type Conversion113/1 -> Relational Operator116/1, Switch115/1
  Data Type Conversion46/1 -> Relational Operator48/1, Switch48/1
  Data Type Conversion63/1 -> Relational Operator65/1, Switch65/1
  Data Type Conversion107/1 -> Relational Operator110/1, Switch110/1
  Constant119/1 -> Data Type Conversion117/1
  Logical Operator43/1 -> Switch45/2
  Logical Operator87/1 -> Switch89/2
  Data Type Conversion97/1 -> Relational Operator99/1, Switch99/1
  [VDDM_5vAPS1OoRCFS_flg] -> Logical Operator/2
  Constant58/1 -> Data Type Conversion60/1
  [DTC_clocker] -> Relational Operator31/2
  Data Type Conversion95/1 -> Relational Operator97/1, Switch97/1
  Switch67/1 -> Switch66/3
  Switch84/1 -> Switch73/3
  Relational Operator87/1 -> Logical Operator85/1
  Constant136/1 -> Logical Operator99/2
  [DTC_clocker] -> Relational Operator118/2
  Switch119/1 -> Switch118/3
  [DTC_clocker] -> Relational Operator83/2
  Relational Operator121/1 -> Logical Operator118/1
  Logical Operator24/1 -> Switch26/2
  Constant70/1 -> Data Type Conversion63/1
  Constant129/1 -> Logical Operator119/2
  Data Type Conversion102/1 -> Relational Operator104/1, Switch106/1
  Relational Operator62/1 -> Logical Operator61/1
  Relational Operator118/1 -> Logical Operator115/1
  Switch91/1 -> Switch90/3
  [VDDM_FrVCUNoComCFS_flg] -> Logical Operator83/2
  Switch113/1 -> Switch112/3
  Logical Operator28/1 -> Switch30/2
  Relational Operator46/1 -> Logical Operator44/1
  Data Type Conversion96/1 -> Relational Operator98/1, Switch98/1
  [DTC_clocker] -> Relational Operator79/2
  Constant42/1 -> Data Type Conversion35/1
  Data Type Conversion118/1 -> Relational Operator121/1, Switch121/1
  Data Type Conversion108/1 -> Relational Operator111/1, Switch111/1
  Constant10/1 -> Data Type Conversion6/1
  Logical Operator80/1 -> Switch72/2
  Relational Operator58/1 -> Logical Operator56/1
  Logical Operator117/1 -> Switch120/2
  Data Type Conversion25/1 -> Relational Operator27/1, Switch27/1
  [VDDM_Lv2ErrCFS_flg] -> Logical Operator46/2
  Relational Operator91/1 -> Logical Operator89/1
  Logical Operator104/1 -> Switch107/2
  Relational Operator21/1 -> Logical Operator19/1
  Switch20/1 -> Switch19/3
  [DTC_clocker] -> Relational Operator44/2
  Logical Operator66/1 -> Switch68/2
  Relational Operator117/1 -> Logical Operator114/1
  [DTC_clocker] -> Relational Operator82/2
  Data Type Conversion77/1 -> Relational Operator79/1, Switch79/1
  Data Type Conversion1/1 -> Relational Operator1/1, Switch2/1
  [VDDM_C3CCU2CSCFS_flg] -> Logical Operator19/2
  Switch61/1 -> Switch60/3
  Switch99/1 -> Switch98/3
  Data Type Conversion37/1 -> Relational Operator39/1, Switch39/1
  Logical Operator89/1 -> Switch91/2
  Constant131/1 -> Logical Operator111/2
  [VDDM_IniLVLoCFS_flg] -> Logical Operator40/2
  Relational Operator61/1 -> Logical Operator59/1
  Logical Operator61/1 -> Switch64/2
  Data Type Conversion110/1 -> Relational Operator103/1, Switch103/1
  Logical Operator79/1 -> Switch81/2
  [VDDM_ZoneDrSigErrCFS_flg] -> Logical Operator84/2
  [DTC_clocker] -> Relational Operator108/2
  Switch111/1 -> Switch110/3
  [DTC_clocker] -> Relational Operator23/2
  Logical Operator91/1 -> Switch94/2
  Logical Operator48/1 -> Switch50/2
  Switch75/1 -> Switch74/3
  Logical Operator25/1 -> Switch27/2
  [VDDM_DCDCEnaCFS_flg] -> Logical Operator24/2
  [DTC_clocker] -> Relational Operator116/2
  [ZoneFrMalfunLevel_enum] -> Logical Operator69/2
  Logical Operator101/1 -> Switch104/2
  [VDDM_APSCorrErrCFS_flg] -> Logical Operator71/2
  Logical Operator96/1 -> Switch98/2
  Switch58/1 -> Switch57/3
  [DTC_clocker] -> Relational Operator24/2
  Data Type Conversion30/1 -> Relational Operator23/1, Switch22/1
  Relational Operator109/1 -> Logical Operator106/1
  [DTC_clocker] -> Relational Operator65/2
  Data Type Conversion59/1 -> Relational Operator61/1, Switch61/1
  Relational Operator47/1 -> Logical Operator45/1
  [VDDM_Lv3ErrCFS_flg] -> Logical Operator47/2
  Logical Operator5/1 -> Switch6/2
  [VDDM_KeyAuthCFS_flg] -> Logical Operator32/2
  [DTC_clocker] -> Relational Operator104/2
  Constant29/1 -> Data Type Conversion22/1
  Constant99/1 -> Data Type Conversion92/1
  Constant121/1 -> Data Type Conversion119/1
  [DTC_clocker] -> Relational Operator120/2
  Constant66/1 -> Data Type Conversion68/1
  Logical Operator115/1 -> Switch118/2
  Relational Operator66/1 -> Logical Operator64/1
  Constant83/1 -> Data Type Conversion71/1
  Data Type Conversion13/1 -> Relational Operator15/1, Switch15/1
  Logical Operator71/1 -> Switch74/2
  [DTC_clocker] -> Relational Operator71/2
  [DTC_clocker] -> Relational Operator96/2
  Constant106/1 -> Data Type Conversion105/1
  [DTC_clocker] -> Relational Operator73/2
  [VDDM_C3CCU1LCCFS_flg] -> Logical Operator17/2
  Data Type Conversion117/1 -> Relational Operator120/1, Switch120/1
  [DTC_clocker] -> Relational Operator57/2
  [DTC_clocker] -> Relational Operator80/2
  Data Type Conversion45/1 -> Relational Operator47/1, Switch47/1
  [VDDM_C3BMS6RCCFS_flg] -> Logical Operator15/2
  Logical Operator118/1 -> Switch121/2
  Relational Operator22/1 -> Logical Operator21/1
  [DTC_clocker] -> Relational Operator105/2
  Logical Operator57/1 -> Switch59/2
  Relational Operator60/1 -> Logical Operator58/1
  Constant97/1 -> Data Type Conversion99/1
  Relational Operator26/1 -> Logical Operator24/1
  Data Type Conversion31/1 -> Relational Operator32/1, Switch34/1
  Switch21/1 -> Switch20/3
  [DTC_clocker] -> Relational Operator2/2
  Constant112/1 -> Data Type Conversion110/1
  Constant113/1 -> Data Type Conversion101/1
  [DTC_clocker] -> Relational Operator109/2
  Data Type Conversion75/1 -> Relational Operator77/1, Switch77/1
  Logical Operator12/1 -> Switch13/2
  [DTC_clocker] -> Relational Operator20/2
  Data Type Conversion67/1 -> Relational Operator69/1, Switch69/1
  Constant103/1 -> Data Type Conversion91/1
  Logical Operator29/1 -> Switch31/2
  Data Type Conversion88/1 -> Relational Operator90/1, Switch90/1
  [DTC_clocker] -> Relational Operator78/2
  [DTC_clocker] -> Relational Operator91/2
  [DTC_clocker] -> Relational Operator35/2
  Relational Operator7/1 -> Logical Operator6/1
  [VDDM_Shifter1RCErrCFS_flg] -> Logical Operator65/2
  Constant142/1 -> Logical Operator112/2
  Constant116/1 -> Data Type Conversion115/1
  Logical Operator51/1 -> Switch54/2
  Relational Operator40/1 -> Logical Operator38/1
  [VDDM_EPB1RCErrCFS_flg] -> Logical Operator93/2
  [VDDM_EPSSigErrCFS_flg] -> Logical Operator89/2
  Relational Operator54/1 -> Logical Operator52/1
  Relational Operator39/1 -> Logical Operator37/1
  Logical Operator42/1 -> Switch43/2
  [DTC_clocker] -> Relational Operator111/2
  Data Type Conversion104/1 -> Relational Operator107/1, Switch107/1
  [VDDM_EPB1NoComCFS_flg] -> Logical Operator91/2
  [VDDM_5vAPS2OoRCFS_flg] -> Logical Operator2/2
  Switch40/1 -> Switch39/3
  Constant111/1 -> Data Type Conversion109/1
  Constant50/1 -> Data Type Conversion43/1
  Logical Operator95/1 -> Switch97/2
  [DTC_clocker] -> Relational Operator102/2
  Logical Operator102/1 -> Switch106/2
  [DTC_clocker] -> Relational Operator90/2
  [DTC_clocker] -> Relational Operator67/2
  Data Type Conversion62/1 -> Relational Operator64/1, Switch63/1
  Data Type Conversion101/1 -> Relational Operator105/1, Switch104/1
  Constant91/1 -> Data Type Conversion84/1
  Logical Operator81/1 -> Switch84/2
  Constant143/1 -> Logical Operator105/2
  Logical Operator108/1 -> Switch111/2
  Constant107/1 -> Data Type Conversion106/1
  Constant104/1 -> Data Type Conversion96/1
  Constant96/1 -> Data Type Conversion98/1
  Switch12/1 -> Switch21/3
  [DTC_clocker] -> Relational Operator115/2
  [DTC_clocker] -> Relational Operator121/2
  Data Type Conversion48/1 -> Relational Operator50/1, Switch50/1
  [VDDM_CCUSigErrCFS_flg] -> Logical Operator78/2
  [VDDM_C3CCU1RCCFS_flg] -> Logical Operator18/2
  Constant150/1 -> Logical Operator103/2
  Logical Operator72/1 -> Switch73/2
  Constant84/1 -> Data Type Conversion76/1
  [DTC_clocker] -> Relational Operator39/2
  Constant109/1 -> Data Type Conversion107/1
  [VDDM_ZoneFrSigErrCFS_flg] -> Logical Operator85/2
  Logical Operator36/1 -> Switch38/2
  Logical Operator106/1 -> Switch109/2
  Constant46/1 -> Data Type Conversion48/1
  Logical Operator99/1 -> Switch101/2
  [VDDM_FRDoorSWCFS_flg] -> Logical Operator35/2
  Relational Operator116/1 -> Logical Operator113/1
  Constant77/1 -> Data Type Conversion79/1
  Logical Operator7/1 -> Switch8/2
  [DTC_clocker] -> Relational Operator22/2
  Constant24/1 -> Data Type Conversion16/1
  Constant86/1 -> Data Type Conversion88/1
  Data Type Conversion120/1 -> Relational Operator113/1, Switch113/1
  Relational Operator106/1 -> Logical Operator103/1
  Relational Operator31/1 -> Logical Operator29/1
  Constant61/1 -> Data Type Conversion54/1
  [VDDM_BrkSWNoBacCFS_flg] -> Logical Operator5/2
  Logical Operator73/1 -> Switch75/2
  Logical Operator50/1 -> Switch42/2
  Data Type Conversion56/1 -> Relational Operator58/1, Switch58/1
  Switch86/1 -> Switch85/3
  [VDDM_LVSupHiCFS_flg] -> Logical Operator43/2
  Switch104/1 -> Switch103/3
  Data Type Conversion89/1 -> Relational Operator91/1, Switch91/1
  Constant114/1 -> Data Type Conversion103/1
  [DTC_clocker] -> Relational Operator3/2
  [DTC_clocker] -> Relational Operator106/2
  Data Type Conversion119/1 -> Relational Operator112/1, Switch112/1
  Constant59/1 -> Data Type Conversion52/1
  Switch85/1 -> Switch84/3
  Switch110/1 -> Switch109/3
  [VDDM_TailgaSWCFS_flg] -> Logical Operator67/2
  [DTC_clocker] -> Relational Operator25/2
  Logical Operator41/1 -> Switch44/2
  Relational Operator3/1 -> Logical Operator1/1
  Logical Operator13/1 -> Switch15/2
  Logical Operator14/1 -> Switch16/2
  Data Type Conversion105/1 -> Relational Operator108/1, Switch108/1
  Switch96/1 -> Switch95/3
  Data Type Conversion64/1 -> Relational Operator66/1, Switch66/1
  Switch66/1 -> Switch65/3
  Constant146/1 -> Logical Operator108/2
  Relational Operator67/1 -> Logical Operator65/1
  Switch95/1 -> Switch94/3
  Switch55/1 -> Switch54/3
  Constant145/1 -> Logical Operator107/2
  Constant35/1 -> Data Type Conversion37/1
  [DTC_clocker] -> Relational Operator110/2
  [VDDM_APS1SigOoRCFS_flg] -> Logical Operator70/2
  Logical Operator116/1 -> Switch119/2
  [DTC_clocker] -> Relational Operator48/2
  Switch117/1 -> Switch116/3
  Switch77/1 -> Switch76/3
  Constant31/1 -> Data Type Conversion24/1
  Constant149/1 -> Logical Operator101/2
  Constant79/1 -> Data Type Conversion72/1
  [DTC_clocker] -> Relational Operator100/2
  Constant108/1 -> Data Type Conversion102/1
  Switch121/1 -> Switch120/3
  Switch103/1 -> Switch102/3
  Data Type Conversion40/1 -> Relational Operator33/1, Switch32/1
  [DTC_clocker] -> Relational Operator119/2
  Relational Operator104/1 -> Logical Operator102/1
  Data Type Conversion85/1 -> Relational Operator87/1, Switch87/1
  Switch72/1 -> Switch81/3
  Constant95/1 -> Data Type Conversion97/1
  Relational Operator56/1 -> Logical Operator54/1
  Logical Operator107/1 -> Switch110/2
  Data Type Conversion36/1 -> Relational Operator38/1, Switch38/1
  [DTC_clocker] -> Relational Operator53/2
  Relational Operator75/1 -> Logical Operator73/1
  Constant135/1 -> Logical Operator98/2
  [VDDM_Shifter1NoComCFS_flg] -> Logical Operator64/2
  Logical Operator110/1 -> Switch103/2
  Relational Operator97/1 -> Logical Operator95/1
  Data Type Conversion90/1 -> Relational Operator83/1, Switch82/1
  Data Type Conversion22/1 -> Relational Operator24/1, Switch23/1
  Constant138/1 -> Logical Operator92/2
  Data Type Conversion116/1 -> Relational Operator119/1, Switch119/1
  Switch4/1 -> Switch3/3
  Constant144/1 -> Logical Operator106/2
  Switch36/1 -> Switch35/3
  [DTC_clocker] -> Relational Operator103/2
  Switch17/1 -> Switch16/3
  Constant139/1 -> Logical Operator102/2
  Switch120/1 -> Switch119/3
  Relational Operator68/1 -> Logical Operator66/1
  [VDDM_C3BMS1RCCFS_flg] -> Logical Operator11/2
  Relational Operator23/1 -> Logical Operator30/1
  Switch98/1 -> Switch97/3
  Relational Operator80/1 -> Logical Operator78/1
  [DTC_clocker] -> Relational Operator34/2
  [DTC_clocker] -> Relational Operator112/2
  Data Type Conversion103/1 -> Relational Operator106/1, Switch105/1
  Switch24/1 -> Switch13/3
  [DTC_clocker] -> Relational Operator18/2
  Logical Operator113/1 -> Switch115/2
  Constant125/1 -> Logical Operator115/2
  [VDDM_C3BMS6CSCFS_flg] -> Logical Operator13/2
  [DTC_clocker] -> Relational Operator117/2
  Switch47/1 -> Switch46/3
  Relational Operator108/1 -> Logical Operator105/1
  Relational Operator42/1 -> Logical Operator41/1
  Data Type Conversion24/1 -> Relational Operator26/1, Switch26/1
  [VDDM_BMSSigErrCFS_flg] -> Logical Operator76/2
  Logical Operator65/1 -> Switch67/2
  [VDDM_MidLvSaChkCFS_flg] -> Logical Operator58/2
  Relational Operator84/1 -> Logical Operator82/1
  Constant127/1 -> Logical Operator117/2
  [DTC_clocker] -> Relational Operator89/2
  [DTC_clocker] -> Relational Operator114/2
  [DTC_clocker] -> Relational Operator9/2
  Data Type Conversion78/1 -> Relational Operator80/1, Switch80/1
  [VDDM_DrVCUNoComCFS_flg] -> Logical Operator81/2
  Constant80/1 -> Data Type Conversion73/1
  Logical Operator8/1 -> Switch9/2
  Data Type Conversion114/1 -> Relational Operator117/1, Switch117/1
  Data Type Conversion5/1 -> Relational Operator6/1, Switch6/1
  Logical Operator67/1 -> Switch69/2
  [DTC_clocker] -> Relational Operator107/2
  Relational Operator79/1 -> Logical Operator77/1
  Switch102/1 -> Switch111/3
  Switch64/1 -> Switch53/3
  Relational Operator8/1 -> Logical Operator7/1
  Constant124/1 -> Data Type Conversion113/1
  Switch25/1 -> Switch24/3
  Constant57/1 -> Data Type Conversion59/1
  Constant120/1 -> Data Type Conversion118/1
  Relational Operator81/1 -> Logical Operator79/1
  [DTC_clocker] -> Relational Operator38/2
  Relational Operator64/1 -> Logical Operator62/1
  [DTC_clocker] -> Relational Operator15/2
  Constant32/1 -> Data Type Conversion25/1
  Relational Operator96/1 -> Logical Operator94/1
  Logical Operator63/1 -> Switch65/2
  Data Type Conversion10/1 -> Relational Operator11/1, Switch11/1
  Constant55/1 -> Data Type Conversion57/1
  Logical Operator112/1 -> Switch116/2
  Data Type Conversion92/1 -> Relational Operator94/1, Switch93/1
  Constant130/1 -> Logical Operator120/2
  Constant132/1 -> Logical Operator113/2
  Relational Operator110/1 -> Logical Operator107/1
  Switch97/1 -> Switch96/3
  Switch76/1 -> Switch75/3
  Constant102/1 -> Data Type Conversion95/1
  [VDDM_FCMACCSigErrCFS_flg] -> Logical Operator77/2
  [VDDM_DrStSWCFS_flg] -> Logical Operator25/2
  Data Type Conversion83/1 -> Relational Operator85/1, Switch85/1
  Constant118/1 -> Data Type Conversion112/1
  [VDDM_Lv4ErrCFS_flg] -> Logical Operator48/2
  Logical Operator15/1 -> Switch17/2
  Constant105/1 -> Data Type Conversion104/1
  Relational Operator115/1 -> Logical Operator111/1
  Data Type Conversion79/1 -> Relational Operator81/1, Switch81/1
  Data Type Conversion115/1 -> Relational Operator118/1, Switch118/1
  [VDDM_Lv1ErrCFS_flg] -> Logical Operator45/2
  Switch93/1 -> Switch92/3
  Data Type Conversion47/1 -> Relational Operator49/1, Switch49/1
  Switch118/1 -> Switch117/3
  Switch116/1 -> Switch105/3
  Relational Operator33/1 -> Logical Operator40/1
  [DTC_clocker] -> Relational Operator55/2
  Constant9/1 -> Data Type Conversion/1
  Relational Operator86/1 -> Logical Operator84/1
  Constant34/1 -> Data Type Conversion26/1
  Relational Operator107/1 -> Logical Operator104/1
  Switch30/1 -> Switch29/3
  [VDDM_ESC1NoComCFS_flg] -> Logical Operator29/2
  Logical Operator38/1 -> Switch40/2
  Logical Operator100/1 -> Switch92/2
  Constant72/1 -> Data Type Conversion65/1
  Switch115/1 -> Switch114/3
  [VDDM_FCM1CSErrCFS_flg] -> Logical Operator75/2
  Constant133/1 -> Switch115/3
  Data Type Conversion99/1 -> Relational Operator101/1, Switch101/1
  [DTC_clocker] -> Relational Operator60/2
  Switch37/1 -> Switch36/3
  [DTC_clocker] -> Relational Operator64/2
  Switch51/1 -> Switch50/3
  Data Type Conversion60/1 -> Relational Operator53/1, Switch52/1
  Logical Operator34/1 -> Switch36/2
  Data Type Conversion9/1 -> Relational Operator10/1, Switch10/1
  Logical Operator84/1 -> Switch86/2
  [VDDM_ACCAccelCmdErrCFS_flg] -> Logical Operator79/2
  Logical Operator56/1 -> Switch58/2
  Switch109/1 -> Switch108/3
  Logical Operator103/1 -> Switch105/2
  Logical Operator18/1 -> Switch20/2
  Constant30/1 -> Data Type Conversion23/1
  Data Type Conversion112/1 -> Relational Operator114/1, Switch116/1
  Constant21/1 -> Data Type Conversion14/1
  Data Type Conversion94/1 -> Relational Operator96/1, Switch96/1
  Relational Operator43/1 -> Logical Operator50/1
  Relational Operator51/1 -> Logical Operator49/1
  Constant148/1 -> Logical Operator110/2
  VDDM_5vAPS1OoRCFS_flg/1 -> [VDDM_5vAPS1OoRCFS_flg]
  VDDM_5vAPS2OoRCFS_flg/1 -> [VDDM_5vAPS2OoRCFS_flg]
  VDDM_BMSRdyCFS_flg/1 -> [VDDM_BMSRdyCFS_flg]
  VDDM_BrkSWErrCFS_flg/1 -> [VDDM_BrkSWErrCFS_flg]
  VDDM_BrkSWNoBacCFS_flg/1 -> [VDDM_BrkSWNoBacCFS_flg]
  VDDM_C1ABM1CSCFS_flg/1 -> [VDDM_C1ABM1CSCFS_flg]
  VDDM_C1ABM1LCCFS_flg/1 -> [VDDM_C1ABM1LCCFS_flg]
  VDDM_C1ABM1RCCFS_flg/1 -> [VDDM_C1ABM1RCCFS_flg]
  VDDM_C3BMS1CSCFS_flg/1 -> [VDDM_C3BMS1CSCFS_flg]
  VDDM_C3BMS1LCCFS_flg/1 -> [VDDM_C3BMS1LCCFS_flg]
  VDDM_C3BMS1RCCFS_flg/1 -> [VDDM_C3BMS1RCCFS_flg]
  VDDM_C3BMS6CSCFS_flg/1 -> [VDDM_C3BMS6CSCFS_flg]
  VDDM_C3BMS6LCCFS_flg/1 -> [VDDM_C3BMS6LCCFS_flg]
  VDDM_C3BMS6RCCFS_flg/1 -> [VDDM_C3BMS6RCCFS_flg]
  VDDM_C3CCU1RCCFS_flg/1 -> [VDDM_C3CCU1RCCFS_flg]
  VDDM_C3CCU1LCCFS_flg/1 -> [VDDM_C3CCU1LCCFS_flg]
  VDDM_C3CCU1CSCFS_flg/1 -> [VDDM_C3CCU1CSCFS_flg]
  VDDM_C3CCU2CSCFS_flg/1 -> [VDDM_C3CCU2CSCFS_flg]
  VDDM_C3CCU2LCCFS_flg/1 -> [VDDM_C3CCU2LCCFS_flg]
  VDDM_C3CCU2RCCFS_flg/1 -> [VDDM_C3CCU2RCCFS_flg]
  VDDM_KeyAuthCFS_flg/1 -> [VDDM_KeyAuthCFS_flg]
  VDDM_IniLVLoCFS_flg/1 -> [VDDM_IniLVLoCFS_flg]
  VDDM_HiLvSaChkCFS_flg/1 -> [VDDM_HiLvSaChkCFS_flg]
  VDDM_HVB4PreCFS_flg/1 -> [VDDM_HVB4PreCFS_flg]
  VDDM_HVRlyCloCFS_flg/1 -> [VDDM_HVRlyCloCFS_flg]
  VDDM_HVRlyOpCFS_flg/1 -> [VDDM_HVRlyOpCFS_flg]
  VDDM_FRDoorSWCFS_flg/1 -> [VDDM_FRDoorSWCFS_flg]
  VDDM_FLDoorSWCFS_flg/1 -> [VDDM_FLDoorSWCFS_flg]
  VDDM_ESC5RCErrCFS_flg/1 -> [VDDM_ESC5RCErrCFS_flg]
  VDDM_ESC5NoComCFS_flg/1 -> [VDDM_ESC5NoComCFS_flg]
  VDDM_ESC5CSErrCFS_flg/1 -> [VDDM_ESC5CSErrCFS_flg]
  VDDM_ESC1RCErrCFS_flg/1 -> [VDDM_ESC1RCErrCFS_flg]
  VDDM_ESC1NoComCFS_flg/1 -> [VDDM_ESC1NoComCFS_flg]
  VDDM_ESC1CSErrCFS_flg/1 -> [VDDM_ESC1CSErrCFS_flg]
  VDDM_EPBUnlockTOCFS_flg/1 -> [VDDM_EPBUnlockTOCFS_flg]
  VDDM_EPBLockTOCFS_flg/1 -> [VDDM_EPBLockTOCFS_flg]
  VDDM_DrStSWCFS_flg/1 -> [VDDM_DrStSWCFS_flg]
  VDDM_DCDCEnaCFS_flg/1 -> [VDDM_DCDCEnaCFS_flg]
  VDDM_DCDCDisCFS_flg/1 -> [VDDM_DCDCDisCFS_flg]
  VDDM_DCDC4PreCFS_flg/1 -> [VDDM_DCDC4PreCFS_flg]
  VDDM_RRDoorSWCFS_flg/1 -> [VDDM_RRDoorSWCFS_flg]
  VDDM_Shifter1CSErrCFS_flg/1 -> [VDDM_Shifter1CSErrCFS_flg]
  VDDM_Shifter1NoComCFS_flg/1 -> [VDDM_Shifter1NoComCFS_flg]
  VDDM_Shifter1RCErrCFS_flg/1 -> [VDDM_Shifter1RCErrCFS_flg]
  VDDM_HoodSWCFS_flg/1 -> [VDDM_HoodSWCFS_flg]
  VDDM_TailgaSWCFS_flg/1 -> [VDDM_TailgaSWCFS_flg]
  VINP_ZoneDrMalfunLevel_enum/1 -> [VINP_ZoneDrMalfunLevel_enum]
  ZoneFrMalfunLevel_enum/1 -> [ZoneFrMalfunLevel_enum]
  VDDM_APS1SigOoRCFS_flg/1 -> [VDDM_APS1SigOoRCFS_flg]
  VDDM_APS2SigOoRCFS_flg/1 -> [VDDM_APS2SigOoRCFS_flg]
  VDDM_APSCorrErrCFS_flg/1 -> [VDDM_APSCorrErrCFS_flg]
  VDDM_FCM1NoComCFS_flg/1 -> [VDDM_FCM1NoComCFS_flg]
  VDDM_FCM1RCErrCFS_flg/1 -> [VDDM_FCM1RCErrCFS_flg]
  VDDM_FCM1CSErrCFS_flg/1 -> [VDDM_FCM1CSErrCFS_flg]
  VDDM_CCUSigErrCFS_flg/1 -> [VDDM_CCUSigErrCFS_flg]
  VDDM_FCMACCSigErrCFS_flg/1 -> [VDDM_FCMACCSigErrCFS_flg]
  VDDM_BMSSigErrCFS_flg/1 -> [VDDM_BMSSigErrCFS_flg]
  VDDM_ACCAccelCmdErrCFS_flg/1 -> [VDDM_ACCAccelCmdErrCFS_flg]
  VDDM_ESCSigErrCFS_flg/1 -> [VDDM_ESCSigErrCFS_flg]
  VDDM_ShifterSigErrCFS_flg/1 -> [VDDM_ShifterSigErrCFS_flg]
  VDDM_RLDoorSWCFS_flg/1 -> [VDDM_RLDoorSWCFS_flg]
  VDDM_ONtoRdyCFS_flg/1 -> [VDDM_ONtoRdyCFS_flg]
  VDDM_OBC4PreCFS_flg/1 -> [VDDM_OBC4PreCFS_flg]
  VDDM_MCUNR1NoComCFS_flg/1 -> [VDDM_MCUNR1NoComCFS_flg]
  VDDM_MCUNR1RCErrCFS_flg/1 -> [VDDM_MCUNR1RCErrCFS_flg]
  VDDM_MidLvSaChkCFS_flg/1 -> [VDDM_MidLvSaChkCFS_flg]
  VDDM_MCUNR1CSErrCFS_flg/1 -> [VDDM_MCUNR1CSErrCFS_flg]
  VDDM_MCUNF1RCErrCFS_flg/1 -> [VDDM_MCUNF1RCErrCFS_flg]
  VDDM_MCUNF1NoComCFS_flg/1 -> [VDDM_MCUNF1NoComCFS_flg]
  VDDM_MCUNF1CSErrCFS_flg/1 -> [VDDM_MCUNF1CSErrCFS_flg]
  VDDM_MCUDisCFS_flg/1 -> [VDDM_MCUDisCFS_flg]
  VDDM_MCUActCFS_flg/1 -> [VDDM_MCUActCFS_flg]
  VDDM_MCU4PreCFS_flg/1 -> [VDDM_MCU4PreCFS_flg]
  VDDM_Lv4ErrCFS_flg/1 -> [VDDM_Lv4ErrCFS_flg]
  VDDM_Lv3ErrCFS_flg/1 -> [VDDM_Lv3ErrCFS_flg]
  VDDM_Lv2ErrCFS_flg/1 -> [VDDM_Lv2ErrCFS_flg]
  VDDM_Lv1ErrCFS_flg/1 -> [VDDM_Lv1ErrCFS_flg]
  VDDM_LVSupLoCFS_flg/1 -> [VDDM_LVSupLoCFS_flg]
  VDDM_LVSupHiCFS_flg/1 -> [VDDM_LVSupHiCFS_flg]
  VDDM_LVInErrCFS_flg/1 -> [VDDM_LVInErrCFS_flg]
  VDDM_RrMCUSigErrCFS_flg/1 -> [VDDM_RrMCUSigErrCFS_flg]
  VDDM_FrMCUSigErrCFS_flg/1 -> [VDDM_FrMCUSigErrCFS_flg]
  VDDM_EPSSigErrCFS_flg/1 -> [VDDM_EPSSigErrCFS_flg]
  VDDM_EPS1CSErrCFS_flg/1 -> [VDDM_EPS1CSErrCFS_flg]
  VDDM_EPS1RCErrCFS_flg/1 -> [VDDM_EPS1RCErrCFS_flg]
  VDDM_EPS1NoComCFS_flg/1 -> [VDDM_EPS1NoComCFS_flg]
  VDDM_ZoneFrSigErrCFS_flg/1 -> [VDDM_ZoneFrSigErrCFS_flg]
  VDDM_ZoneDrSigErrCFS_flg/1 -> [VDDM_ZoneDrSigErrCFS_flg]
  VDDM_FrVCUNoComCFS_flg/1 -> [VDDM_FrVCUNoComCFS_flg]
  VDDM_DrVCUNoComCFS_flg/1 -> [VDDM_DrVCUNoComCFS_flg]
  VDDM_EPB1NoComCFS_flg/1 -> [VDDM_EPB1NoComCFS_flg]
  VDDM_EPB1RCErrCFS_flg/1 -> [VDDM_EPB1RCErrCFS_flg]
  VDDM_EPB1CSErrCFS_flg/1 -> [VDDM_EPB1CSErrCFS_flg]
  VDDM_EPBSigErrCFS_flg/1 -> [VDDM_EPBSigErrCFS_flg]
  VDDM_FrMCUNTqErrCFS_flg/1 -> [VDDM_FrMCUNTqErrCFS_flg]
  VDDM_RrMCUNTqErrCFS_flg/1 -> [VDDM_RrMCUNTqErrCFS_flg]
  [VDDM_DTCDetect_enum] -> VDDM_DTCDetect_enum/1
